simulink model "RocketSEDynamic"  (R2017b)
settings: Solver=VariableStepAuto  StartTime=0.0  StopTime=10.0  RelTol=1e-3
values from neighbouring files (symbols this model uses):
  Ad = expm(A*T)    [KalmanBSP.m]    (also in ReadARISData.m = expm(A*Tau); SEFromData.m = expm(A*Tau); SEFromDataWithGPS.m = expm(A*Tau); SEFromDataWithPressure.m = expm(A*Tau))
  B = [0;0;0]    [KalmanBSP.m]    (also in ReadARISData.m = [0;0;0;0;0]; SEFromData.m = [0;0;0;0;0]; SEFromDataWithGPS.m; SEFromDataWithPressure.m = [0;0;0;0;0;0])
  C = [1 0 0;0 0 1]    [KalmanBSP.m]    (also in ReadARISData.m = [1 0 0 0 0; 0 0 1 -1 0;0 0 0 0 1]; SEFromData.m = [1 0 0 0 0; SEFromDataWithGPS.m; SEFromDataWithPressure.m = [0 0 1 0 0 0;0 0 0 1 0 0;0 0 0 1 0 0;0 0 0 0 1 0])
  D = [0;0]    [KalmanBSP.m]    (also in ReadARISData.m = [0]; SEFromData.m = [0]; SEFromDataWithGPS.m; SEFromDataWithPressure.m)
  P0 = 1013.25    [PressureFunction.m]    (also in SEFromData.m = eye(6); SEFromDataWithGPS.m = eye(); SEFromDataWithPressure.m = eye(6); SEFromDataWithPressureGPS.m = eye(6))
  R = 8.314    [CalcPressure.m]    (also in KalmanBSP.m = [varp 0;0 vara]; ReadARISData.m = diag([2^32;MACL;2^32]); SEFromData.m = diag([GPSvar ACLvar BM1var BM2var TRMvar]); SEFromDataWithGPS.m = diag([GPSvar ACLvar]))
  Tau = TimeVec(k)-TimeVec(k-1)    [ReadARISData.m]    (also in SEFromData.m = TimeVec(end)/length(TimeVec); SEFromDataWithGPS.m = TimeVec(end)/length(TimeVec); SEFromDataWithPressure.m = TimeVec(end)/length(TimeVec); SEFromDataWithPressureGPS.m = TimeVec(end)/length(TimeVec))
  Time = 0:0.001:30    [KalmanBSP.m]
  x = Ad*x + B*u(k)    [KalmanBSP.m]    (also in ReadARISData.m = x + K*([Height;acc_mes(k);Temp] - C*x); SEFromData.m = Ad*x + Bd*u(k); SEFromDataWithGPS.m = Ad*x + Bd*u(k); SEFromDataWithPressure.m = Ad*x + Bd*u(k))
undefined symbols (not defined in the file or in its folder): Discrete
libraries: ctrlSharedLib x1
settings Model: Creator=geilomat  LastModifiedBy=geilomat

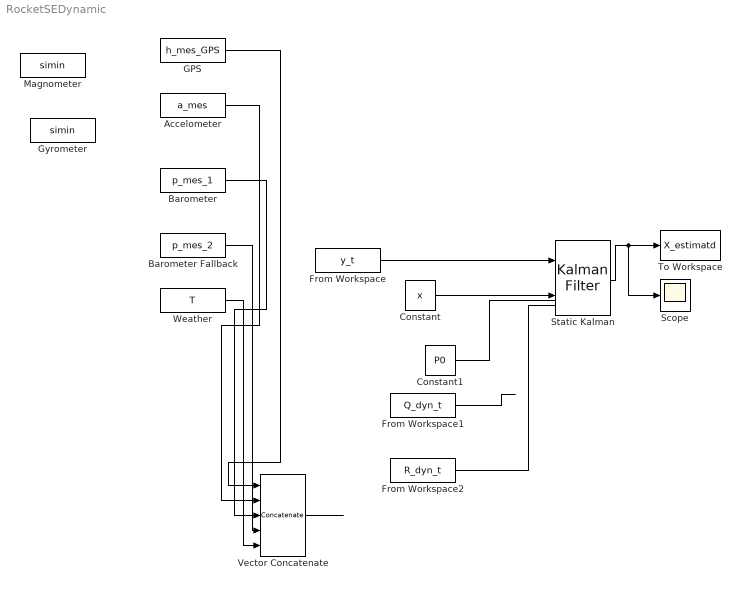
== system RocketSEDynamic ==
  Accelometer : FromWorkspace  VariableName=a_mes  SampleTime=0
  "Barometer " : FromWorkspace  VariableName=p_mes_1  SampleTime=0
  "Barometer Fallback " : FromWorkspace  VariableName=p_mes_2  SampleTime=0
  Constant : Constant  Value=x
  Constant1 : Constant  Value=P0
  From Workspace : FromWorkspace  VariableName=y_t  SampleTime=Tau  Interpolate=off  OutputAfterFinalValue=Holding final value
  From Workspace1 : FromWorkspace  VariableName=Q_dyn_t  SampleTime=Tau
  From Workspace2 : FromWorkspace  VariableName=R_dyn_t  SampleTime=Tau
  "GPS " : FromWorkspace  VariableName=h_mes_GPS  SampleTime=Tau  Interpolate=off  OutputAfterFinalValue=Holding final value
  "Gyrometer " : FromWorkspace  VariableName=simin  SampleTime=0
  "Magnometer " : FromWorkspace  VariableName=simin  SampleTime=0
  Scope : Scope
  Static Kalman : ctrlSharedLib/Kalman Filter  TimeDomain=Discrete-Time  UseCurrentEstimator=on  ModelSource=Individual A, B, C, D matrices  ModelSourceVariable=ss(0.95,1,1,0,1)  A=Ad  B=B  C=C  D=D  NumberOfStates=1  NumberOfInputs=1  NumberOfOutputs=1  InitialEstimateSource=Input port  X0=0  P0=10  UseK=off  UseGH=off  NumberOfProcessNoiseInputs=1  G=1  TimeInvariantG=on  H=0  TimeInvariantH=on  Q=Q  TimeInvariantQ=on  R=R  TimeInvariantR=on  N=0  TimeInvariantN=on  AddInputPort=off  AddEnablePort=off  OutputEstimatedY=off  OutputP=off  Ts=-1
      settings: SourceProductBaseCode=CT
  To Workspace : ToWorkspace  VariableName=X_estimatd  SaveFormat=Structure With Time  SampleTime=-1
  Vector Concatenate : Concatenate  NumInputs=5  Mode=Multidimensional array  ConcatenateDimension=3
  "Weather " : FromWorkspace  VariableName=T  SampleTime=0
  wires:
  "Barometer "/1 -> Vector Concatenate/3
  From Workspace1/1 -> ?
  Accelometer/1 -> Vector Concatenate/2
  "Weather "/1 -> Vector Concatenate/5
  "Barometer Fallback "/1 -> Vector Concatenate/4
  "GPS "/1 -> Vector Concatenate/1
  Constant/1 -> Static Kalman/2
  Static Kalman/1 -> To Workspace/1, Scope/1
  Constant1/1 -> ?
  From Workspace2/1 -> ?
  From Workspace/1 -> Static Kalman/1
  Vector Concatenate/1 -> ?
